simulink model "zadanieWSimulinku"  (R2024a)
settings: Solver=ode4  StartTime=0.0  StopTime=9  FixedStep=0.001  RelTol=1e-3
undefined symbols (not defined in the file): A, B, b1, b2, C, D, k1, k2, m1, m2
settings Model: Creator=adasf  LastModifiedBy=adasf

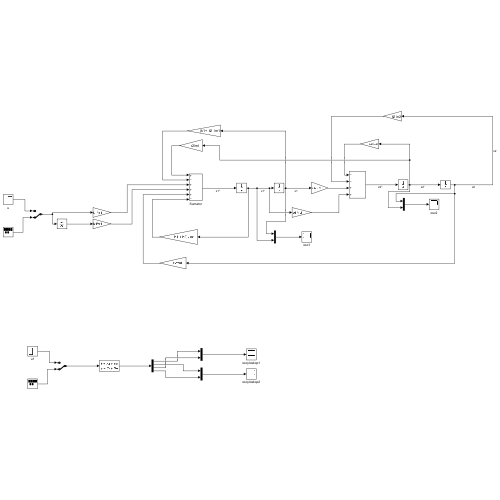
[thumbnail: Simulink's stored preview of the top-level diagram]
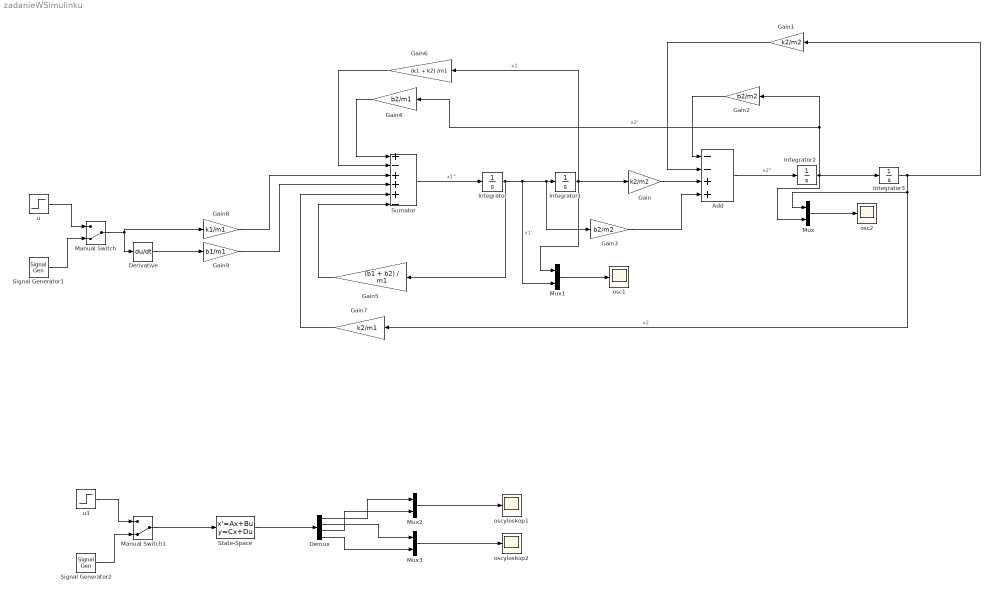
== system zadanieWSimulinku ==
  Add : Sum  Inputs=--++
  Demux : Demux
  Derivative : Derivative
  Gain : Gain  Gain=k2/m2
  Gain1 : Gain  Gain=k2/m2
  Gain2 : Gain  Gain=b2/m2
  Gain3 : Gain  Gain=b2/m2
  Gain4 : Gain  Gain=b2/m1
  Gain5 : Gain  Gain=(b1 + b2) / m1
  Gain6 : Gain  Gain=(k1 + k2) /m1
  Gain7 : Gain  Gain=k2/m1
  Gain8 : Gain  Gain=k1/m1
  Gain9 : Gain  Gain=b1/m1
  Integrator{,1..3} (4 alike) : Integrator
  Manual Switch : ManualSwitch  CurrentSetting=0
  Manual Switch1 : ManualSwitch  CurrentSetting=0
  Mux{,1..3} (4 alike) : Mux  Inputs=2
  Signal Generator1 : SignalGenerator  WaveForm=square  Amplitude=0.1  Frequency=1.53  Units=rad/sec
  Signal Generator2 : SignalGenerator  WaveForm=square  Amplitude=0.1  Frequency=1.53  Units=rad/sec
  State-Space : StateSpace  A=A  B=B  C=C  D=D  InitialCondition=0
  Sumator : Sum  Inputs=+-+++-
  osc1 : Scope
  osc2 : Scope
  oscyloskop1 : Scope
  oscyloskop2 : Scope
  u : Step  Before=1  SampleTime=0
  u1 : Step  Before=1  SampleTime=1
  wires:
  Sumator/1 -> Integrator/1  "x1\""
  Integrator/1 -> Mux1/2, Gain3/1, Integrator1/1, Gain5/1  "x1'"
  Integrator1/1 -> Mux1/1, Gain/1, Gain6/1  "x1"
  Gain/1 -> Add/3
  Integrator2/1 -> Mux/2, Integrator3/1, Gain4/1, Gain2/1  "x2'"
  Add/1 -> Integrator2/1  "x2\""
  Integrator3/1 -> Gain7/1, Mux/1, Gain1/1  "x2"
  u/1 -> Manual Switch/1
  Signal Generator1/1 -> Manual Switch/2
  Gain1/1 -> Add/2
  Gain2/1 -> Add/1
  Gain3/1 -> Add/4
  Gain4/1 -> Sumator/1
  Gain5/1 -> Sumator/6
  Gain6/1 -> Sumator/2
  Gain7/1 -> Sumator/5
  Manual Switch/1 -> Derivative/1, Gain8/1
  Derivative/1 -> Gain9/1
  Gain8/1 -> Sumator/3
  Gain9/1 -> Sumator/4
  Mux/1 -> osc2/1
  Mux1/1 -> osc1/1
  u1/1 -> Manual Switch1/1
  Signal Generator2/1 -> Manual Switch1/2
  Manual Switch1/1 -> State-Space/1
  State-Space/1 -> Demux/1
  Demux/1 -> Mux2/1
  Demux/4 -> Mux3/2
  Mux2/1 -> oscyloskop1/1
  Mux3/1 -> oscyloskop2/1
  Demux/3 -> Mux2/2
  Demux/2 -> Mux3/1
